simulink model "afe_dq_inv_3L_psm"  (R2025a)
settings: Solver=ode1be  StartTime=0.0  StopTime=simlength  FixedStep=tc  MaxStep=tc
undefined symbols (not defined in the file): Adrso, Amplitude_U, Amplitude_V, Amplitude_W, b, Crso, CTRPIFF_CLIP_RELEASE, dead_time_AFE, dead_time_INV, deepNEGeta, deepNEGxi, deepPOSxi, emf_fb_p, emf_fb_p_ccaller_1, emf_fb_p_ccaller_2, emf_p, emf_p_ccaller_1, emf_p_ccaller_2, end_time_LVRT, fPWM_AFE, fPWM_INV, g0_500Hz, g1_500Hz, ibez, id_lim, Igrid_phase_normalization_factor, iq_lim, ixi_pos_ref_lim, Jm, kg, ki_afe, ki_i, ki_rc_grid, ki_vs, ki_w, kp_afe, kp_i, kp_rc_grid, kp_vs, kp_w, kw, Ld_norm, Ldrso, Lq_norm, Ls_norm, magnitude, motorc_m_scale, n1, n10, omega_bez, omega_grid_emulator_nom, omega_grid_nom, omega_m_bez, omega_m_sim, Phase_shift, pll_i1, pll_i1_ddsrt, pll_p, pll_p_ddsrt, pll_p_frt ... (+28)
libraries: fl_lib x159, nesl_utility x86, cstblocks x14, single_phase_transformer_lib x3, threephase_inductor_lib x2, simulink x2, flexshaft_lib x1, pmsm_uvw_with_harmonics_lib x1
(part 4 of 9)

== system afe_dq_inv_3L_psm/afe_dq_inv_psm_mod1/afe/dclink_measure/R_derating ==
  Step : Step  After=107.4e3/2  SampleTime=0
  Step1 : Step  Time=1.1  After=-107.4e3/2  SampleTime=0
  Sum : Sum  Inputs=|++
  DR : Outport
  wires:
  Step1/1 -> Sum/2
  Step/1 -> Sum/1
  Sum/1 -> DR/1

== system afe_dq_inv_3L_psm/afe_dq_inv_psm_mod1/afe/sv_pwm/modulator1 ==
  u : Inport
  v : Inport  Port=2
  w : Inport  Port=3
  phase : Inport  Port=4
  Bus Creator : BusCreator  Inputs=3
  PWM generator u : Subsystem  mask{f=fPWM_AFE, m_up=1, m_low=-1, dead_time=dead_time_AFE, pos_cmd_gate=15, neg_cmd_gate=-10, polarity=1}
      mask prompts: f "Frequency (Hz)"; m_up "Max Input Modulation Value"; m_low "Min Input Modulation Value"; dead_time "Dead Time (s)"; pos_cmd_gate "Positive Gate Voltage (V)"; neg_cmd_gate "Negative Gate Voltage (V)"; polarity "Polarity (pu)"
  PWM generator v : Subsystem  mask{f=fPWM_AFE, m_up=1, m_low=-1, dead_time=dead_time_AFE, pos_cmd_gate=15, neg_cmd_gate=-10, polarity=1}
      mask prompts: f "Frequency (Hz)"; m_up "Max Input Modulation Value"; m_low "Min Input Modulation Value"; dead_time "Dead Time (s)"; pos_cmd_gate "Positive Gate Voltage (V)"; neg_cmd_gate "Negative Gate Voltage (V)"; polarity "Polarity (pu)"
  PWM generator w : Subsystem  mask{f=fPWM_AFE, m_up=1, m_low=-1, dead_time=dead_time_AFE, pos_cmd_gate=15, neg_cmd_gate=-10, polarity=1}
      mask prompts: f "Frequency (Hz)"; m_up "Max Input Modulation Value"; m_low "Min Input Modulation Value"; dead_time "Dead Time (s)"; pos_cmd_gate "Positive Gate Voltage (V)"; neg_cmd_gate "Negative Gate Voltage (V)"; polarity "Polarity (pu)"
  cmd_gates : Outport
  wires:
  u/1 -> PWM generator u/1(m)
  w/1 -> PWM generator w/1(m)
  v/1 -> PWM generator v/1(m)
  phase/1 -> PWM generator w/2(phase), PWM generator v/2(phase), PWM generator u/2(phase)
  PWM generator v/1(mv) -> Bus Creator/2  "PWM generator v"
  PWM generator u/1(mu) -> Bus Creator/1  "PWM generator u"
  PWM generator w/1(mw) -> Bus Creator/3  "PWM generator w"
  Bus Creator/1 -> cmd_gates/1

== system afe_dq_inv_3L_psm/afe_dq_inv_psm_mod1/afe/three-level-inverter_ttype/switch_1 ==
  Capacitor : fl_lib/Electrical/Electrical Elements/Capacitor  c=Csnubber F  r=Rsnubber Ohm  g=0 1/Ohm  i_specify=off  i_priority=None  i=0 A  i_nominal_specify=off  i_nominal_value=1  i_nominal_unit=A  v_specify=off  v_priority=None  v=0 V  v_nominal_specify=off  v_nominal_value=1  v_nominal_unit=V  vc_specify=off  vc_priority=High  vc=0 V  vc_nominal_specify=off  vc_nominal_value=1  vc_nominal_unit=V
  Diode : fl_lib/Electrical/Electrical Elements/Diode  Vf=Vdon_diode V  Ron=Rdon_diode Ohm  Goff=1e-8 1/Ohm  i_specify=off  i_priority=None  i=0 A  i_nominal_specify=off  i_nominal_value=1  i_nominal_unit=A  v_specify=off  v_priority=None  v=0 V  v_nominal_specify=off  v_nominal_value=1  v_nominal_unit=V
  Switch : fl_lib/Electrical/Electrical Elements/Switch  R_closed=Ron Ohm  G_open=1e-8 1/Ohm  Threshold=7.5  i_specify=off  i_priority=None  i=0 A  i_nominal_specify=off  i_nominal_value=1  i_nominal_unit=A  v_specify=off  v_priority=None  v=0 V  v_nominal_specify=off  v_nominal_value=1  v_nominal_unit=V
  G : PMIOPort  Side=Left
  C : PMIOPort  Port=2  Side=Left
  E : PMIOPort  Port=3  Side=Right
  connections:
  C/RConn1 -- Capacitor/LConn1 -- Diode/RConn1 -- Switch/RConn2
  Switch/RConn1 -- G/RConn1
  Switch/LConn1 -- E/RConn1 -- Capacitor/RConn1 -- Diode/LConn1

== system afe_dq_inv_3L_psm/afe_dq_inv_psm_mod1/afe/three-level-inverter_ttype/switch_10 ==
  Capacitor : fl_lib/Electrical/Electrical Elements/Capacitor  c=Csnubber F  r=Rsnubber Ohm  g=0 1/Ohm  i_specify=off  i_priority=None  i=0 A  i_nominal_specify=off  i_nominal_value=1  i_nominal_unit=A  v_specify=off  v_priority=None  v=0 V  v_nominal_specify=off  v_nominal_value=1  v_nominal_unit=V  vc_specify=off  vc_priority=High  vc=0 V  vc_nominal_specify=off  vc_nominal_value=1  vc_nominal_unit=V
  Diode : fl_lib/Electrical/Electrical Elements/Diode  Vf=Vdon_diode V  Ron=Rdon_diode Ohm  Goff=1e-8 1/Ohm  i_specify=off  i_priority=None  i=0 A  i_nominal_specify=off  i_nominal_value=1  i_nominal_unit=A  v_specify=off  v_priority=None  v=0 V  v_nominal_specify=off  v_nominal_value=1  v_nominal_unit=V
  Switch : fl_lib/Electrical/Electrical Elements/Switch  R_closed=Ron Ohm  G_open=1e-8 1/Ohm  Threshold=7.5  i_specify=off  i_priority=None  i=0 A  i_nominal_specify=off  i_nominal_value=1  i_nominal_unit=A  v_specify=off  v_priority=None  v=0 V  v_nominal_specify=off  v_nominal_value=1  v_nominal_unit=V
  G : PMIOPort  Side=Left
  C : PMIOPort  Port=2  Side=Left
  E : PMIOPort  Port=3  Side=Right
  connections:
  Capacitor/RConn1 -- Diode/LConn1 -- E/RConn1 -- Switch/LConn1
  Switch/RConn1 -- G/RConn1
  Capacitor/LConn1 -- Diode/RConn1 -- Switch/RConn2 -- C/RConn1

== system afe_dq_inv_3L_psm/afe_dq_inv_psm_mod1/afe/three-level-inverter_ttype/switch_11 ==
  Capacitor : fl_lib/Electrical/Electrical Elements/Capacitor  c=Csnubber F  r=Rsnubber Ohm  g=0 1/Ohm  i_specify=off  i_priority=None  i=0 A  i_nominal_specify=off  i_nominal_value=1  i_nominal_unit=A  v_specify=off  v_priority=None  v=0 V  v_nominal_specify=off  v_nominal_value=1  v_nominal_unit=V  vc_specify=off  vc_priority=High  vc=0 V  vc_nominal_specify=off  vc_nominal_value=1  vc_nominal_unit=V
  Diode : fl_lib/Electrical/Electrical Elements/Diode  Vf=Vdon_diode V  Ron=Rdon_diode Ohm  Goff=1e-8 1/Ohm  i_specify=off  i_priority=None  i=0 A  i_nominal_specify=off  i_nominal_value=1  i_nominal_unit=A  v_specify=off  v_priority=None  v=0 V  v_nominal_specify=off  v_nominal_value=1  v_nominal_unit=V
  Switch : fl_lib/Electrical/Electrical Elements/Switch  R_closed=Ron Ohm  G_open=1e-8 1/Ohm  Threshold=7.5  i_specify=off  i_priority=None  i=0 A  i_nominal_specify=off  i_nominal_value=1  i_nominal_unit=A  v_specify=off  v_priority=None  v=0 V  v_nominal_specify=off  v_nominal_value=1  v_nominal_unit=V
  G : PMIOPort  Side=Left
  C : PMIOPort  Port=2  Side=Left
  E : PMIOPort  Port=3  Side=Right
  connections:
  C/RConn1 -- Switch/RConn2 -- Diode/RConn1 -- Capacitor/LConn1
  Switch/RConn1 -- G/RConn1
  Switch/LConn1 -- E/RConn1 -- Diode/LConn1 -- Capacitor/RConn1

== system afe_dq_inv_3L_psm/afe_dq_inv_psm_mod1/afe/three-level-inverter_ttype/switch_12 ==
  Capacitor : fl_lib/Electrical/Electrical Elements/Capacitor  c=Csnubber F  r=Rsnubber Ohm  g=0 1/Ohm  i_specify=off  i_priority=None  i=0 A  i_nominal_specify=off  i_nominal_value=1  i_nominal_unit=A  v_specify=off  v_priority=None  v=0 V  v_nominal_specify=off  v_nominal_value=1  v_nominal_unit=V  vc_specify=off  vc_priority=High  vc=0 V  vc_nominal_specify=off  vc_nominal_value=1  vc_nominal_unit=V
  Diode : fl_lib/Electrical/Electrical Elements/Diode  Vf=Vdon_diode V  Ron=Rdon_diode Ohm  Goff=1e-8 1/Ohm  i_specify=off  i_priority=None  i=0 A  i_nominal_specify=off  i_nominal_value=1  i_nominal_unit=A  v_specify=off  v_priority=None  v=0 V  v_nominal_specify=off  v_nominal_value=1  v_nominal_unit=V
  Switch : fl_lib/Electrical/Electrical Elements/Switch  R_closed=Ron Ohm  G_open=1e-8 1/Ohm  Threshold=7.5  i_specify=off  i_priority=None  i=0 A  i_nominal_specify=off  i_nominal_value=1  i_nominal_unit=A  v_specify=off  v_priority=None  v=0 V  v_nominal_specify=off  v_nominal_value=1  v_nominal_unit=V
  G : PMIOPort  Side=Left
  C : PMIOPort  Port=2  Side=Left
  E : PMIOPort  Port=3  Side=Right
  connections:
  Capacitor/RConn1 -- Diode/LConn1 -- E/RConn1 -- Switch/LConn1
  Switch/RConn1 -- G/RConn1
  Capacitor/LConn1 -- Diode/RConn1 -- Switch/RConn2 -- C/RConn1

== system afe_dq_inv_3L_psm/afe_dq_inv_psm_mod1/afe/three-level-inverter_ttype/switch_2 ==
  Capacitor : fl_lib/Electrical/Electrical Elements/Capacitor  c=Csnubber F  r=Rsnubber Ohm  g=0 1/Ohm  i_specify=off  i_priority=None  i=0 A  i_nominal_specify=off  i_nominal_value=1  i_nominal_unit=A  v_specify=off  v_priority=None  v=0 V  v_nominal_specify=off  v_nominal_value=1  v_nominal_unit=V  vc_specify=off  vc_priority=High  vc=0 V  vc_nominal_specify=off  vc_nominal_value=1  vc_nominal_unit=V
  Diode : fl_lib/Electrical/Electrical Elements/Diode  Vf=Vdon_diode V  Ron=Rdon_diode Ohm  Goff=1e-8 1/Ohm  i_specify=off  i_priority=None  i=0 A  i_nominal_specify=off  i_nominal_value=1  i_nominal_unit=A  v_specify=off  v_priority=None  v=0 V  v_nominal_specify=off  v_nominal_value=1  v_nominal_unit=V
  Switch : fl_lib/Electrical/Electrical Elements/Switch  R_closed=Ron Ohm  G_open=1e-8 1/Ohm  Threshold=7.5  i_specify=off  i_priority=None  i=0 A  i_nominal_specify=off  i_nominal_value=1  i_nominal_unit=A  v_specify=off  v_priority=None  v=0 V  v_nominal_specify=off  v_nominal_value=1  v_nominal_unit=V
  G : PMIOPort  Side=Left
  C : PMIOPort  Port=2  Side=Left
  E : PMIOPort  Port=3  Side=Right
  connections:
  Capacitor/RConn1 -- Diode/LConn1 -- E/RConn1 -- Switch/LConn1
  Switch/RConn1 -- G/RConn1
  Capacitor/LConn1 -- Diode/RConn1 -- Switch/RConn2 -- C/RConn1

== system afe_dq_inv_3L_psm/afe_dq_inv_psm_mod1/afe/three-level-inverter_ttype/switch_3 ==
  Capacitor : fl_lib/Electrical/Electrical Elements/Capacitor  c=Csnubber F  r=Rsnubber Ohm  g=0 1/Ohm  i_specify=off  i_priority=None  i=0 A  i_nominal_specify=off  i_nominal_value=1  i_nominal_unit=A  v_specify=off  v_priority=None  v=0 V  v_nominal_specify=off  v_nominal_value=1  v_nominal_unit=V  vc_specify=off  vc_priority=High  vc=0 V  vc_nominal_specify=off  vc_nominal_value=1  vc_nominal_unit=V
  Diode : fl_lib/Electrical/Electrical Elements/Diode  Vf=Vdon_diode V  Ron=Rdon_diode Ohm  Goff=1e-8 1/Ohm  i_specify=off  i_priority=None  i=0 A  i_nominal_specify=off  i_nominal_value=1  i_nominal_unit=A  v_specify=off  v_priority=None  v=0 V  v_nominal_specify=off  v_nominal_value=1  v_nominal_unit=V
  Switch : fl_lib/Electrical/Electrical Elements/Switch  R_closed=Ron Ohm  G_open=1e-8 1/Ohm  Threshold=7.5  i_specify=off  i_priority=None  i=0 A  i_nominal_specify=off  i_nominal_value=1  i_nominal_unit=A  v_specify=off  v_priority=None  v=0 V  v_nominal_specify=off  v_nominal_value=1  v_nominal_unit=V
  G : PMIOPort  Side=Left
  C : PMIOPort  Port=2  Side=Left
  E : PMIOPort  Port=3  Side=Right
  connections:
  C/RConn1 -- Switch/RConn2 -- Diode/RConn1 -- Capacitor/LConn1
  Switch/RConn1 -- G/RConn1
  Switch/LConn1 -- E/RConn1 -- Diode/LConn1 -- Capacitor/RConn1

== system afe_dq_inv_3L_psm/afe_dq_inv_psm_mod1/afe/three-level-inverter_ttype/switch_4 ==
  Capacitor : fl_lib/Electrical/Electrical Elements/Capacitor  c=Csnubber F  r=Rsnubber Ohm  g=0 1/Ohm  i_specify=off  i_priority=None  i=0 A  i_nominal_specify=off  i_nominal_value=1  i_nominal_unit=A  v_specify=off  v_priority=None  v=0 V  v_nominal_specify=off  v_nominal_value=1  v_nominal_unit=V  vc_specify=off  vc_priority=High  vc=0 V  vc_nominal_specify=off  vc_nominal_value=1  vc_nominal_unit=V
  Diode : fl_lib/Electrical/Electrical Elements/Diode  Vf=Vdon_diode V  Ron=Rdon_diode Ohm  Goff=1e-8 1/Ohm  i_specify=off  i_priority=None  i=0 A  i_nominal_specify=off  i_nominal_value=1  i_nominal_unit=A  v_specify=off  v_priority=None  v=0 V  v_nominal_specify=off  v_nominal_value=1  v_nominal_unit=V
  Switch : fl_lib/Electrical/Electrical Elements/Switch  R_closed=Ron Ohm  G_open=1e-8 1/Ohm  Threshold=7.5  i_specify=off  i_priority=None  i=0 A  i_nominal_specify=off  i_nominal_value=1  i_nominal_unit=A  v_specify=off  v_priority=None  v=0 V  v_nominal_specify=off  v_nominal_value=1  v_nominal_unit=V
  G : PMIOPort  Side=Left
  C : PMIOPort  Port=2  Side=Left
  E : PMIOPort  Port=3  Side=Right
  connections:
  Capacitor/RConn1 -- Diode/LConn1 -- E/RConn1 -- Switch/LConn1
  Switch/RConn1 -- G/RConn1
  Capacitor/LConn1 -- Diode/RConn1 -- Switch/RConn2 -- C/RConn1

== system afe_dq_inv_3L_psm/afe_dq_inv_psm_mod1/afe/three-level-inverter_ttype/switch_5 ==
  Capacitor : fl_lib/Electrical/Electrical Elements/Capacitor  c=Csnubber F  r=Rsnubber Ohm  g=0 1/Ohm  i_specify=off  i_priority=None  i=0 A  i_nominal_specify=off  i_nominal_value=1  i_nominal_unit=A  v_specify=off  v_priority=None  v=0 V  v_nominal_specify=off  v_nominal_value=1  v_nominal_unit=V  vc_specify=off  vc_priority=High  vc=0 V  vc_nominal_specify=off  vc_nominal_value=1  vc_nominal_unit=V
  Diode : fl_lib/Electrical/Electrical Elements/Diode  Vf=Vdon_diode V  Ron=Rdon_diode Ohm  Goff=1e-8 1/Ohm  i_specify=off  i_priority=None  i=0 A  i_nominal_specify=off  i_nominal_value=1  i_nominal_unit=A  v_specify=off  v_priority=None  v=0 V  v_nominal_specify=off  v_nominal_value=1  v_nominal_unit=V
  Switch : fl_lib/Electrical/Electrical Elements/Switch  R_closed=Ron Ohm  G_open=1e-8 1/Ohm  Threshold=7.5  i_specify=off  i_priority=None  i=0 A  i_nominal_specify=off  i_nominal_value=1  i_nominal_unit=A  v_specify=off  v_priority=None  v=0 V  v_nominal_specify=off  v_nominal_value=1  v_nominal_unit=V
  G : PMIOPort  Side=Left
  C : PMIOPort  Port=2  Side=Left
  E : PMIOPort  Port=3  Side=Right
  connections:
  C/RConn1 -- Switch/RConn2 -- Diode/RConn1 -- Capacitor/LConn1
  Switch/RConn1 -- G/RConn1
  Switch/LConn1 -- E/RConn1 -- Diode/LConn1 -- Capacitor/RConn1

== system afe_dq_inv_3L_psm/afe_dq_inv_psm_mod1/afe/three-level-inverter_ttype/switch_6 ==
  Capacitor : fl_lib/Electrical/Electrical Elements/Capacitor  c=Csnubber F  r=Rsnubber Ohm  g=0 1/Ohm  i_specify=off  i_priority=None  i=0 A  i_nominal_specify=off  i_nominal_value=1  i_nominal_unit=A  v_specify=off  v_priority=None  v=0 V  v_nominal_specify=off  v_nominal_value=1  v_nominal_unit=V  vc_specify=off  vc_priority=High  vc=0 V  vc_nominal_specify=off  vc_nominal_value=1  vc_nominal_unit=V
  Diode : fl_lib/Electrical/Electrical Elements/Diode  Vf=Vdon_diode V  Ron=Rdon_diode Ohm  Goff=1e-8 1/Ohm  i_specify=off  i_priority=None  i=0 A  i_nominal_specify=off  i_nominal_value=1  i_nominal_unit=A  v_specify=off  v_priority=None  v=0 V  v_nominal_specify=off  v_nominal_value=1  v_nominal_unit=V
  Switch : fl_lib/Electrical/Electrical Elements/Switch  R_closed=Ron Ohm  G_open=1e-8 1/Ohm  Threshold=7.5  i_specify=off  i_priority=None  i=0 A  i_nominal_specify=off  i_nominal_value=1  i_nominal_unit=A  v_specify=off  v_priority=None  v=0 V  v_nominal_specify=off  v_nominal_value=1  v_nominal_unit=V
  G : PMIOPort  Side=Left
  C : PMIOPort  Port=2  Side=Left
  E : PMIOPort  Port=3  Side=Right
  connections:
  Capacitor/RConn1 -- Diode/LConn1 -- E/RConn1 -- Switch/LConn1
  Switch/RConn1 -- G/RConn1
  Capacitor/LConn1 -- Diode/RConn1 -- Switch/RConn2 -- C/RConn1

== system afe_dq_inv_3L_psm/afe_dq_inv_psm_mod1/afe/three-level-inverter_ttype/switch_7 ==
  Capacitor : fl_lib/Electrical/Electrical Elements/Capacitor  c=Csnubber F  r=Rsnubber Ohm  g=0 1/Ohm  i_specify=off  i_priority=None  i=0 A  i_nominal_specify=off  i_nominal_value=1  i_nominal_unit=A  v_specify=off  v_priority=None  v=0 V  v_nominal_specify=off  v_nominal_value=1  v_nominal_unit=V  vc_specify=off  vc_priority=High  vc=0 V  vc_nominal_specify=off  vc_nominal_value=1  vc_nominal_unit=V
  Diode : fl_lib/Electrical/Electrical Elements/Diode  Vf=Vdon_diode V  Ron=Rdon_diode Ohm  Goff=1e-8 1/Ohm  i_specify=off  i_priority=None  i=0 A  i_nominal_specify=off  i_nominal_value=1  i_nominal_unit=A  v_specify=off  v_priority=None  v=0 V  v_nominal_specify=off  v_nominal_value=1  v_nominal_unit=V
  Switch : fl_lib/Electrical/Electrical Elements/Switch  R_closed=Ron Ohm  G_open=1e-8 1/Ohm  Threshold=7.5  i_specify=off  i_priority=None  i=0 A  i_nominal_specify=off  i_nominal_value=1  i_nominal_unit=A  v_specify=off  v_priority=None  v=0 V  v_nominal_specify=off  v_nominal_value=1  v_nominal_unit=V
  G : PMIOPort  Side=Left
  C : PMIOPort  Port=2  Side=Left
  E : PMIOPort  Port=3  Side=Right
  connections:
  C/RConn1 -- Switch/RConn2 -- Diode/RConn1 -- Capacitor/LConn1
  Switch/RConn1 -- G/RConn1
  Switch/LConn1 -- E/RConn1 -- Diode/LConn1 -- Capacitor/RConn1

== system afe_dq_inv_3L_psm/afe_dq_inv_psm_mod1/afe/three-level-inverter_ttype/switch_8 ==
  Capacitor : fl_lib/Electrical/Electrical Elements/Capacitor  c=Csnubber F  r=Rsnubber Ohm  g=0 1/Ohm  i_specify=off  i_priority=None  i=0 A  i_nominal_specify=off  i_nominal_value=1  i_nominal_unit=A  v_specify=off  v_priority=None  v=0 V  v_nominal_specify=off  v_nominal_value=1  v_nominal_unit=V  vc_specify=off  vc_priority=High  vc=0 V  vc_nominal_specify=off  vc_nominal_value=1  vc_nominal_unit=V
  Diode : fl_lib/Electrical/Electrical Elements/Diode  Vf=Vdon_diode V  Ron=Rdon_diode Ohm  Goff=1e-8 1/Ohm  i_specify=off  i_priority=None  i=0 A  i_nominal_specify=off  i_nominal_value=1  i_nominal_unit=A  v_specify=off  v_priority=None  v=0 V  v_nominal_specify=off  v_nominal_value=1  v_nominal_unit=V
  Switch : fl_lib/Electrical/Electrical Elements/Switch  R_closed=Ron Ohm  G_open=1e-8 1/Ohm  Threshold=7.5  i_specify=off  i_priority=None  i=0 A  i_nominal_specify=off  i_nominal_value=1  i_nominal_unit=A  v_specify=off  v_priority=None  v=0 V  v_nominal_specify=off  v_nominal_value=1  v_nominal_unit=V
  G : PMIOPort  Side=Left
  C : PMIOPort  Port=2  Side=Left
  E : PMIOPort  Port=3  Side=Right
  connections:
  Capacitor/RConn1 -- Diode/LConn1 -- E/RConn1 -- Switch/LConn1
  Switch/RConn1 -- G/RConn1
  Capacitor/LConn1 -- Diode/RConn1 -- Switch/RConn2 -- C/RConn1

== system afe_dq_inv_3L_psm/afe_dq_inv_psm_mod1/afe/three-level-inverter_ttype/switch_9 ==
  Capacitor : fl_lib/Electrical/Electrical Elements/Capacitor  c=Csnubber F  r=Rsnubber Ohm  g=0 1/Ohm  i_specify=off  i_priority=None  i=0 A  i_nominal_specify=off  i_nominal_value=1  i_nominal_unit=A  v_specify=off  v_priority=None  v=0 V  v_nominal_specify=off  v_nominal_value=1  v_nominal_unit=V  vc_specify=off  vc_priority=High  vc=0 V  vc_nominal_specify=off  vc_nominal_value=1  vc_nominal_unit=V
  Diode : fl_lib/Electrical/Electrical Elements/Diode  Vf=Vdon_diode V  Ron=Rdon_diode Ohm  Goff=1e-8 1/Ohm  i_specify=off  i_priority=None  i=0 A  i_nominal_specify=off  i_nominal_value=1  i_nominal_unit=A  v_specify=off  v_priority=None  v=0 V  v_nominal_specify=off  v_nominal_value=1  v_nominal_unit=V
  Switch : fl_lib/Electrical/Electrical Elements/Switch  R_closed=Ron Ohm  G_open=1e-8 1/Ohm  Threshold=7.5  i_specify=off  i_priority=None  i=0 A  i_nominal_specify=off  i_nominal_value=1  i_nominal_unit=A  v_specify=off  v_priority=None  v=0 V  v_nominal_specify=off  v_nominal_value=1  v_nominal_unit=V
  G : PMIOPort  Side=Left
  C : PMIOPort  Port=2  Side=Left
  E : PMIOPort  Port=3  Side=Right
  connections:
  C/RConn1 -- Switch/RConn2 -- Diode/RConn1 -- Capacitor/LConn1
  Switch/RConn1 -- G/RConn1
  Switch/LConn1 -- E/RConn1 -- Diode/LConn1 -- Capacitor/RConn1

== system afe_dq_inv_3L_psm/afe_dq_inv_psm_mod1/afe_control/current_ctrl/current_transformation ==
  is_a_pu : Inport
  is_b_pu : Inport  Port=2
  is_c_pu : Inport  Port=3
  Bus Creator : BusCreator  Inputs=3
  alphabeta2xieta : MATLAB Function  TreatAsAtomicUnit=on  SystemSampleTime=ts_afe
  uvw2alphabeta : MATLAB Function  TreatAsAtomicUnit=on  SystemSampleTime=ts_afe
  tag scope: is_abc_pu=global, is_eta_pu=global, is_xi_pu=global
  wires:
  is_c_pu/1 -> Bus Creator/3, uvw2alphabeta/3(w)
  alphabeta2xieta/2(eta) -> [is_eta_pu]  "ieta_pu"
  alphabeta2xieta/1(xi) -> [is_xi_pu]  "ixi_pu"
  is_b_pu/1 -> Bus Creator/2, uvw2alphabeta/2(v)
  uvw2alphabeta/2(beta) -> alphabeta2xieta/2(beta)  "ibeta_pu"
  uvw2alphabeta/1(alpha) -> alphabeta2xieta/1(alpha)  "ialpha_pu"
  [gamma_grid_pll] -> alphabeta2xieta/3(gamma)
  is_a_pu/1 -> Bus Creator/1, uvw2alphabeta/1(u)
  Bus Creator/1 -> [is_abc_pu]

== system afe_dq_inv_3L_psm/afe_dq_inv_psm_mod1/afe_control/current_ctrl/rc_current_ctrl ==
  i_grid_eta_ref : Inport
  i_grid_eta : Inport  Port=2
  Gain : Gain  Gain=-1
  pi_eta_rc_grid : Subsystem  mask{kp=kp_rc_grid, ki=ki_rc_grid, ts=ts_afe, sat_pos=1, sat_neg=-1}
  is_eta_ref : Outport
  wires:
  i_grid_eta_ref/1 -> pi_eta_rc_grid/2(ig_eta_ref)  "i_grid_eta_ref"
  i_grid_eta/1 -> pi_eta_rc_grid/1(ig_eta)  "i_grid_eta"
  pi_eta_rc_grid/1(is_eta_ref) -> Gain/1
  Gain/1 -> is_eta_ref/1

== system afe_dq_inv_3L_psm/afe_dq_inv_psm_mod1/afe_control/current_ctrl/sample_hold_normalization ==
  is_a : Inport
  is_b : Inport  Port=2
  is_c : Inport  Port=3
  Gain : Gain  Gain=1/Igrid_phase_normalization_factor
  Gain1 : Gain  Gain=1/Igrid_phase_normalization_factor
  Gain2 : Gain  Gain=1/Igrid_phase_normalization_factor
  Quantizer : Quantizer  QuantizationInterval=CurrentQuantization
  Quantizer1 : Quantizer  QuantizationInterval=CurrentQuantization
  Quantizer2 : Quantizer  QuantizationInterval=CurrentQuantization
  Unit Delay : UnitDelay  SampleTime=ts_afe  HasFrameUpgradeWarning=on
  Unit Delay1 : UnitDelay  SampleTime=ts_afe  HasFrameUpgradeWarning=on
  Unit Delay2 : UnitDelay  SampleTime=ts_afe  HasFrameUpgradeWarning=on
  Zero-Order Hold : ZeroOrderHold  SampleTime=ts_afe
  Zero-Order Hold1 : ZeroOrderHold  SampleTime=ts_afe
  Zero-Order Hold2 : ZeroOrderHold  SampleTime=ts_afe
  is_a_pu : Outport
  is_b_pu : Outport  Port=2
  is_c_pu : Outport  Port=3
  wires:
  is_a/1 -> Quantizer/1
  Unit Delay/1 -> Gain/1
  Zero-Order Hold/1 -> Unit Delay/1
  is_c/1 -> Quantizer2/1
  is_b/1 -> Quantizer1/1
  Gain/1 -> is_a_pu/1
  Gain1/1 -> is_b_pu/1
  Gain2/1 -> is_c_pu/1
  Unit Delay1/1 -> Gain1/1
  Unit Delay2/1 -> Gain2/1
  Zero-Order Hold1/1 -> Unit Delay1/1
  Zero-Order Hold2/1 -> Unit Delay2/1
  Quantizer/1 -> Zero-Order Hold/1
  Quantizer1/1 -> Zero-Order Hold1/1
  Quantizer2/1 -> Zero-Order Hold2/1

== system afe_dq_inv_3L_psm/afe_dq_inv_psm_mod1/afe_control/current_ctrl/xieta_pi_with_vector_antiwindup ==
  is_xi_ref : Inport
  is_xi : Inport  Port=2
  is_eta_ref : Inport  Port=3
  is_eta : Inport  Port=4
  i_eta/i_eta_ref : Scope  NumInputPorts=2
      settings: SampleTime=ts_afe  ActiveDisplayYMinimum=-0.29872  ActiveDisplayYMaximum=0.32463  DataLoggingVariableName=ScopeData2
  i_xi/i_xi_ref : Scope  NumInputPorts=2
      settings: SampleTime=ts_afe  ActiveDisplayYMinimum=-3.84394  ActiveDisplayYMaximum=3.92699
  xieta_vector_pi : Subsystem
  uxi : Outport
  ueta : Outport  Port=2
  wires:
  is_xi/1 -> i_xi/i_xi_ref/1, xieta_vector_pi/1(ixi)  "i_xi"
  is_xi_ref/1 -> i_xi/i_xi_ref/2, xieta_vector_pi/2(ixi_ref)  "i_xi_ref"
  is_eta/1 -> i_eta/i_eta_ref/1, xieta_vector_pi/3(ieta)  "i_eta"
  is_eta_ref/1 -> i_eta/i_eta_ref/2, xieta_vector_pi/4(ieta_ref)  "i_eta_ref"
  xieta_vector_pi/1(uxi) -> uxi/1
  xieta_vector_pi/2(ueta) -> ueta/1

== system afe_dq_inv_3L_psm/afe_dq_inv_psm_mod1/afe_control/grid_current_sampling_and_alpha_beta_transformation/sample_hold_normalization ==
  ig_a : Inport
  ig_b : Inport  Port=2
  ig_c : Inport  Port=3
  Gain : Gain  Gain=1/Igrid_phase_normalization_factor
  Gain1 : Gain  Gain=1/Igrid_phase_normalization_factor
  Gain2 : Gain  Gain=1/Igrid_phase_normalization_factor
  Quantizer : Quantizer  QuantizationInterval=adc_quantization
  Quantizer1 : Quantizer  QuantizationInterval=adc_quantization
  Quantizer2 : Quantizer  QuantizationInterval=adc_quantization
  Unit Delay : UnitDelay  SampleTime=ts_afe  HasFrameUpgradeWarning=on
  Unit Delay1 : UnitDelay  SampleTime=ts_afe  HasFrameUpgradeWarning=on
  Unit Delay2 : UnitDelay  SampleTime=ts_afe  HasFrameUpgradeWarning=on
  Zero-Order Hold : ZeroOrderHold  SampleTime=ts_afe
  Zero-Order Hold1 : ZeroOrderHold  SampleTime=ts_afe
  Zero-Order Hold2 : ZeroOrderHold  SampleTime=ts_afe
  ig_a_pu : Outport
  ig_b_pu : Outport  Port=2
  ig_c_pu : Outport  Port=3
  wires:
  ig_a/1 -> Gain/1
  Zero-Order Hold/1 -> Unit Delay/1
  ig_c/1 -> Gain2/1
  ig_b/1 -> Gain1/1
  Unit Delay/1 -> ig_a_pu/1
  Unit Delay1/1 -> ig_b_pu/1
  Unit Delay2/1 -> ig_c_pu/1
  Zero-Order Hold1/1 -> Unit Delay1/1
  Zero-Order Hold2/1 -> Unit Delay2/1
  Quantizer/1 -> Zero-Order Hold/1
  Gain1/1 -> Quantizer1/1
  Gain2/1 -> Quantizer2/1
  Gain/1 -> Quantizer/1
  Quantizer1/1 -> Zero-Order Hold1/1
  Quantizer2/1 -> Zero-Order Hold2/1

== system afe_dq_inv_3L_psm/afe_dq_inv_psm_mod1/afe_control/grid_voltage_phase_lock_loops/DDSRF-PLL ==
  pll_stageA : Subsystem
  pll_stageB : Subsystem
  gamma_grid_ddsrf_pll : Outport
  omega_grid_ddsrf_pll : Outport  Port=2
  wires:
  pll_stageB/1(gamma_grid_ddsrf_pll) -> pll_stageA/1(gamma_grid), gamma_grid_ddsrf_pll/1
  pll_stageA/2(u_grid_pos_eta) -> pll_stageB/2(u_grid_pos_eta)  "u_grid_pos_eta"
  pll_stageA/1(u_grid_pos_xi) -> pll_stageB/1(u_grid_pos_xi)  "u_grid_pos_xi"
  pll_stageB/2(omega_grid_ddsrf_pll) -> omega_grid_ddsrf_pll/1

== system afe_dq_inv_3L_psm/afe_dq_inv_psm_mod1/afe_control/grid_voltage_phase_lock_loops/DQ-PLL ==
  pll_stageA : Subsystem
  pll_stageB : Subsystem
  gamma_grid_dqpll : Outport
  omega_grid_dqpll : Outport  Port=2
  wires:
  pll_stageA/2(u_grid_pos_eta) -> pll_stageB/2(u_grid_pos_eta)  "u_grid_pos_eta"
  pll_stageB/1(gamma_grid_dqpll) -> pll_stageA/1(gamma_grid), gamma_grid_dqpll/1
  pll_stageA/1(u_grid_pos_xi) -> pll_stageB/1(u_grid_pos_xi)  "u_grid_pos_xi"
  pll_stageB/2(omega_grid_dqpll) -> omega_grid_dqpll/1

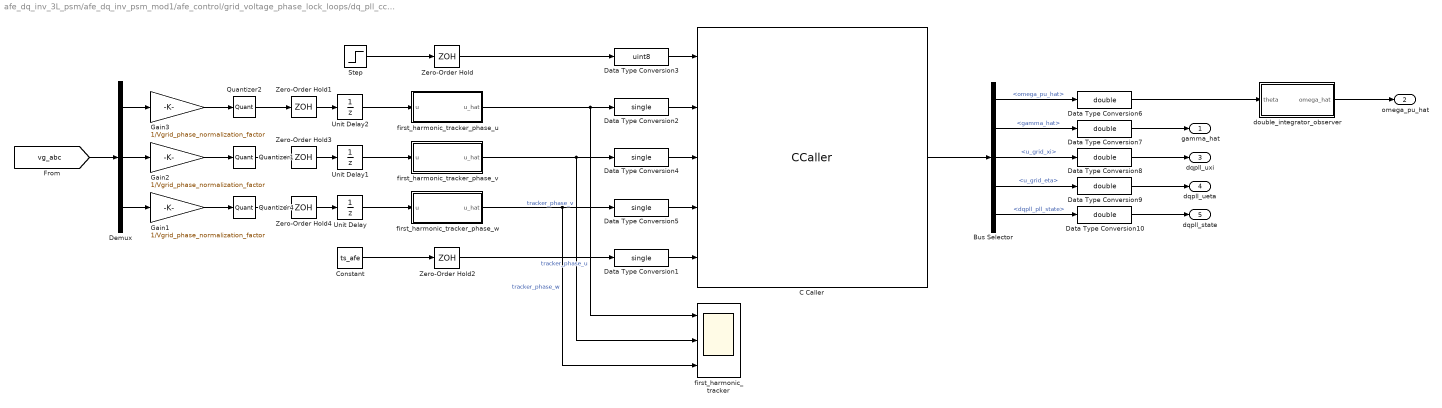
== system afe_dq_inv_3L_psm/afe_dq_inv_psm_mod1/afe_control/grid_voltage_phase_lock_loops/dq_pll_ccaller ==
  Bus Selector : BusSelector  OutputSignals=omega_pu_hat,gamma_hat,u_grid_xi,u_grid_eta,dqpll_pll_state
  C Caller : CCaller  FunctionName=dqpll_grid_process_simulink  PortSpecificationStruct="%)30     .    N H   8    (     @         %    \"     8    !     0         %  0 \"0    $    _    07)G3F%M90  4&]R=$YA;64 4V-O<&4     26YD97@     5'EP90      4VEZ90      27-';&]B86P   X    P    !@    @    $          4    (     0    ,    !         !   P!O=70 #@   #     &    \"     0         !0    @    !     P    $         $  # &]U=  .    .     8    (    !          %    \"     $    &     0         0   ...(+3319 chars)"  SampleTime=ts_afe
  Constant : Constant  Value=ts_afe
  Data Type Conversion{1..2,4..5} (4 alike) : DataTypeConversion  OutDataTypeStr=single  SaturateOnIntegerOverflow=off  RndMeth=Floor
  Data Type Conversion{6..10} (5 alike) : DataTypeConversion  OutDataTypeStr=double  SaturateOnIntegerOverflow=off  RndMeth=Floor
  Data Type Conversion3 : DataTypeConversion  OutDataTypeStr=uint8  SaturateOnIntegerOverflow=off  RndMeth=Floor
  Demux : Demux  Outputs=3
  Gain1 : Gain  Gain=1/Vgrid_phase_normalization_factor
  Gain2 : Gain  Gain=1/Vgrid_phase_normalization_factor
  Gain3 : Gain  Gain=1/Vgrid_phase_normalization_factor
  Quantizer1 : Quantizer  QuantizationInterval=adc_quantization
  Quantizer2 : Quantizer  QuantizationInterval=adc_quantization
  Quantizer4 : Quantizer  QuantizationInterval=adc_quantization
  Step : Step  Time=0.01  Before=1  After=0  SampleTime=0
  Unit Delay : UnitDelay  SampleTime=ts_afe  HasFrameUpgradeWarning=on
  Unit Delay1 : UnitDelay  SampleTime=ts_afe  HasFrameUpgradeWarning=on
  Unit Delay2 : UnitDelay  SampleTime=ts_afe  HasFrameUpgradeWarning=on
  Zero-Order Hold : ZeroOrderHold  SampleTime=ts_afe
  Zero-Order Hold1 : ZeroOrderHold  SampleTime=-1
  Zero-Order Hold2 : ZeroOrderHold  SampleTime=ts_afe
  Zero-Order Hold3 : ZeroOrderHold  SampleTime=-1
  Zero-Order Hold4 : ZeroOrderHold  SampleTime=-1
  double_integrator_observer : Subsystem
  first_harmonic_tracker : Scope  NumInputPorts=3
      settings: SampleTime=ts_afe  ActiveDisplayYMinimum=-1.8039357215166092  ActiveDisplayYMaximum=1.5758593827486038
  first_harmonic_tracker_phase_u : Subsystem
  first_harmonic_tracker_phase_v : Subsystem
  first_harmonic_tracker_phase_w : Subsystem
  gamma_hat : Outport  VectorParamsAs1DForOutWhenUnconnected=off
  omega_pu_hat : Outport  Port=2  VectorParamsAs1DForOutWhenUnconnected=off
  dqpll_uxi : Outport  Port=3  VectorParamsAs1DForOutWhenUnconnected=off
  dqpll_ueta : Outport  Port=4  VectorParamsAs1DForOutWhenUnconnected=off
  dqpll_state : Outport  Port=5  VectorParamsAs1DForOutWhenUnconnected=off
  wires:
  Zero-Order Hold/1 -> Data Type Conversion3/1
  Step/1 -> Zero-Order Hold/1
  Zero-Order Hold2/1 -> Data Type Conversion1/1
  Constant/1 -> Zero-Order Hold2/1
  Data Type Conversion3/1 -> C Caller/1
  Data Type Conversion2/1 -> C Caller/2
  Data Type Conversion4/1 -> C Caller/3
  Data Type Conversion5/1 -> C Caller/4
  Data Type Conversion1/1 -> C Caller/5
  C Caller/1 -> Bus Selector/1
  Bus Selector/1 -> Data Type Conversion6/1  "<omega_pu_hat>"
  Bus Selector/2 -> Data Type Conversion7/1  "<gamma_hat>"
  Bus Selector/3 -> Data Type Conversion8/1  "<u_grid_xi>"
  Bus Selector/4 -> Data Type Conversion9/1  "<u_grid_eta>"
  Bus Selector/5 -> Data Type Conversion10/1  "<dqpll_pll_state>"
  Data Type Conversion6/1 -> double_integrator_observer/1(theta)
  Data Type Conversion7/1 -> gamma_hat/1
  Data Type Conversion10/1 -> dqpll_state/1
  Data Type Conversion8/1 -> dqpll_uxi/1
  Data Type Conversion9/1 -> dqpll_ueta/1
  [vg_abc] -> Demux/1
  Quantizer4/1 -> Zero-Order Hold4/1
  Quantizer2/1 -> Zero-Order Hold1/1
  Gain2/1 -> Quantizer1/1
  Gain3/1 -> Quantizer2/1
  Gain1/1 -> Quantizer4/1
  Zero-Order Hold1/1 -> Unit Delay2/1
  Unit Delay2/1 -> first_harmonic_tracker_phase_u/1(u)
  Demux/1 -> Gain3/1
  Unit Delay1/1 -> first_harmonic_tracker_phase_v/1(u)
  Demux/2 -> Gain2/1
  Demux/3 -> Gain1/1
  Unit Delay/1 -> first_harmonic_tracker_phase_w/1(u)
  Quantizer1/1 -> Zero-Order Hold3/1
  Zero-Order Hold3/1 -> Unit Delay1/1
  Zero-Order Hold4/1 -> Unit Delay/1
  double_integrator_observer/1(omega_hat) -> omega_pu_hat/1
  first_harmonic_tracker_phase_u/1(u_hat) -> first_harmonic_tracker/1, Data Type Conversion2/1  "tracker_phase_u"
  first_harmonic_tracker_phase_v/1(u_hat) -> first_harmonic_tracker/2, Data Type Conversion4/1  "tracker_phase_v"
  first_harmonic_tracker_phase_w/1(u_hat) -> first_harmonic_tracker/3, Data Type Conversion5/1  "tracker_phase_w"

== system afe_dq_inv_3L_psm/afe_dq_inv_psm_mod1/afe_control/grid_voltage_sampling_and_alpha_beta_transformation/sample_hold_normalization ==
  vg_a : Inport
  vg_b : Inport  Port=2
  vg_c : Inport  Port=3
  Gain : Gain  Gain=1/Vgrid_phase_normalization_factor
  Gain1 : Gain  Gain=1/Vgrid_phase_normalization_factor
  Gain2 : Gain  Gain=1/Vgrid_phase_normalization_factor
  Quantizer1 : Quantizer  QuantizationInterval=adc_quantization
  Quantizer2 : Quantizer  QuantizationInterval=adc_quantization
  Quantizer3 : Quantizer  QuantizationInterval=adc_quantization
  Unit Delay : UnitDelay  SampleTime=ts_afe  HasFrameUpgradeWarning=on
  Unit Delay1 : UnitDelay  SampleTime=ts_afe  HasFrameUpgradeWarning=on
  Unit Delay2 : UnitDelay  SampleTime=ts_afe  HasFrameUpgradeWarning=on
  Zero-Order Hold : ZeroOrderHold  SampleTime=ts_afe
  Zero-Order Hold1 : ZeroOrderHold  SampleTime=ts_afe
  Zero-Order Hold2 : ZeroOrderHold  SampleTime=ts_afe
  vg_a_pu : Outport
  vg_b_pu : Outport  Port=2
  vg_c_pu : Outport  Port=3
  wires:
  vg_a/1 -> Gain/1
  Zero-Order Hold/1 -> Unit Delay/1
  vg_c/1 -> Gain2/1
  vg_b/1 -> Gain1/1
  Unit Delay/1 -> vg_a_pu/1
  Unit Delay1/1 -> vg_b_pu/1
  Unit Delay2/1 -> vg_c_pu/1
  Zero-Order Hold1/1 -> Unit Delay1/1
  Zero-Order Hold2/1 -> Unit Delay2/1
  Quantizer1/1 -> Zero-Order Hold/1
  Gain1/1 -> Quantizer2/1
  Gain2/1 -> Quantizer3/1
  Gain/1 -> Quantizer1/1
  Quantizer2/1 -> Zero-Order Hold1/1
  Quantizer3/1 -> Zero-Order Hold2/1

== system afe_dq_inv_3L_psm/afe_dq_inv_psm_mod1/afe_control/islanding_mode_detector/Moving Average Filter ==
  u_7th : Inport
  In3 : Inport  Port=2
  Bus Selector : BusSelector  OutputSignals=ts,sshort,slong,pinput,cbpointer,cbsample,mavg_output
  C Caller : CCaller  FunctionName=mavgflt_process_simulink  PortSpecificationStruct="%)30     .    B H   8    (     @         %    \"     8    !     0         %  0 \"0    $    _    07)G3F%M90  4&]R=$YA;64 4V-O<&4     26YD97@     5'EP90      4VEZ90      27-';&]B86P   X    P    !@    @    $          4    (     0    ,    !         !   P!O=70 #@   #     &    \"     0         !0    @    !     P    $         $  # &]U=  .    .     8    (    !          %    \"     $    &     0         0   ...(+3251 chars)"  SampleTime=ts_afe
  Compare To Zero : simulink/Logic and Bit Operations/Compare To Zero  relop=>  OutDataTypeStr=boolean
  Constant : Constant  Value=9
  Constant5 : Constant  Value=ts_afe
  Data Type Conversion : DataTypeConversion  OutDataTypeStr=single  SaturateOnIntegerOverflow=off  RndMeth=Floor
  Data Type Conversion1 : DataTypeConversion  OutDataTypeStr=single  SaturateOnIntegerOverflow=off  RndMeth=Floor
  Data Type Conversion2 : DataTypeConversion  OutDataTypeStr=single  SaturateOnIntegerOverflow=off  RndMeth=Floor
  Data Type Conversion3 : DataTypeConversion  OutDataTypeStr=double  SaturateOnIntegerOverflow=off  RndMeth=Floor
  Data Type Conversion4 : DataTypeConversion  OutDataTypeStr=uint8  SaturateOnIntegerOverflow=off  RndMeth=Floor
  Data Type Conversion5 : DataTypeConversion  OutDataTypeStr=uint8  SaturateOnIntegerOverflow=off  RndMeth=Floor
  Enabled Subsystem : Subsystem  TreatAsAtomicUnit=on
  Reset Trigger : Subsystem
  Terminator{,1..5} (6 alike) : Terminator
  Zero-Order Hold1 : ZeroOrderHold  SampleTime=ts_afe
  Zero-Order Hold2 : ZeroOrderHold  SampleTime=ts_afe
  xi : Outport
  wires:
  Bus Selector/5 -> Terminator2/1  "<cbpointer>"
  Bus Selector/4 -> Terminator1/1  "<pinput>"
  Data Type Conversion3/1 -> xi/1  "output"
  Zero-Order Hold2/1 -> Data Type Conversion/1  "d1"
  Enabled Subsystem/1(Out1) -> Data Type Conversion1/1
  Compare To Zero/1 -> Enabled Subsystem/Enable
  In3/1 -> Enabled Subsystem/1(In1), Compare To Zero/1  "omega_grid"
  Constant5/1 -> Zero-Order Hold1/1
  Zero-Order Hold1/1 -> Data Type Conversion2/1  "d1"
  Bus Selector/3 -> Terminator4/1  "<slong>"
  Bus Selector/2 -> Terminator3/1  "<sshort>"
  Bus Selector/1 -> Terminator/1  "<ts>"
  C Caller/1 -> Bus Selector/1  "out"
  u_7th/1 -> Zero-Order Hold2/1  "input"
  Data Type Conversion4/1 -> C Caller/5
  Data Type Conversion/1 -> C Caller/1  "input"
  Data Type Conversion5/1 -> C Caller/4
  Data Type Conversion2/1 -> C Caller/3
  Data Type Conversion1/1 -> C Caller/2
  Reset Trigger/1(Out1) -> Data Type Conversion5/1
  Constant/1 -> Data Type Conversion4/1
  Bus Selector/6 -> Terminator5/1  "<cbsample>"
  Bus Selector/7 -> Data Type Conversion3/1  "<mavg_output>"

== system afe_dq_inv_3L_psm/afe_dq_inv_psm_mod1/afe_control/islanding_mode_detector/Moving Average Filter1 ==
  u_7th : Inport
  In3 : Inport  Port=2
  Bus Selector : BusSelector  OutputSignals=ts,sshort,slong,pinput,cbpointer,cbsample,mavg_output
  C Caller : CCaller  FunctionName=mavgflt_process_simulink  PortSpecificationStruct="%)30     .    B H   8    (     @         %    \"     8    !     0         %  0 \"0    $    _    07)G3F%M90  4&]R=$YA;64 4V-O<&4     26YD97@     5'EP90      4VEZ90      27-';&]B86P   X    P    !@    @    $          4    (     0    ,    !         !   P!O=70 #@   #     &    \"     0         !0    @    !     P    $         $  # &]U=  .    .     8    (    !          %    \"     $    &     0         0   ...(+3251 chars)"  SampleTime=ts_afe
  Compare To Zero : simulink/Logic and Bit Operations/Compare To Zero  relop=>  OutDataTypeStr=boolean
  Constant : Constant  Value=10
  Constant5 : Constant  Value=ts_afe
  Data Type Conversion : DataTypeConversion  OutDataTypeStr=single  SaturateOnIntegerOverflow=off  RndMeth=Floor
  Data Type Conversion1 : DataTypeConversion  OutDataTypeStr=single  SaturateOnIntegerOverflow=off  RndMeth=Floor
  Data Type Conversion2 : DataTypeConversion  OutDataTypeStr=single  SaturateOnIntegerOverflow=off  RndMeth=Floor
  Data Type Conversion3 : DataTypeConversion  OutDataTypeStr=double  SaturateOnIntegerOverflow=off  RndMeth=Floor
  Data Type Conversion4 : DataTypeConversion  OutDataTypeStr=uint8  SaturateOnIntegerOverflow=off  RndMeth=Floor
  Data Type Conversion5 : DataTypeConversion  OutDataTypeStr=uint8  SaturateOnIntegerOverflow=off  RndMeth=Floor
  Enabled Subsystem : Subsystem  TreatAsAtomicUnit=on
  Reset Trigger : Subsystem
  Terminator{,1..5} (6 alike) : Terminator
  Zero-Order Hold1 : ZeroOrderHold  SampleTime=ts_afe
  Zero-Order Hold2 : ZeroOrderHold  SampleTime=ts_afe
  xi : Outport
  wires:
  Bus Selector/7 -> Data Type Conversion3/1  "<mavg_output>"
  Bus Selector/6 -> Terminator5/1  "<cbsample>"
  Constant/1 -> Data Type Conversion4/1
  Reset Trigger/1(Out1) -> Data Type Conversion5/1
  Data Type Conversion1/1 -> C Caller/2
  Data Type Conversion2/1 -> C Caller/3
  Data Type Conversion5/1 -> C Caller/4
  Data Type Conversion/1 -> C Caller/1  "input"
  Data Type Conversion4/1 -> C Caller/5
  u_7th/1 -> Zero-Order Hold2/1  "input"
  C Caller/1 -> Bus Selector/1  "out"
  Bus Selector/1 -> Terminator/1  "<ts>"
  Bus Selector/2 -> Terminator3/1  "<sshort>"
  Bus Selector/3 -> Terminator4/1  "<slong>"
  Zero-Order Hold1/1 -> Data Type Conversion2/1  "d1"
  Constant5/1 -> Zero-Order Hold1/1
  In3/1 -> Compare To Zero/1, Enabled Subsystem/1(In1)  "omega_grid"
  Compare To Zero/1 -> Enabled Subsystem/Enable
  Enabled Subsystem/1(Out1) -> Data Type Conversion1/1
  Zero-Order Hold2/1 -> Data Type Conversion/1  "d1"
  Data Type Conversion3/1 -> xi/1  "output"
  Bus Selector/4 -> Terminator1/1  "<pinput>"
  Bus Selector/5 -> Terminator2/1  "<cbpointer>"
